simulink model "CompareBasisMRAC_knownDynamics_Obsolete"  (R2022b)
settings: Solver=ode4  StartTime=0.0  StopTime=30  FixedStep=1e-3  RelTol=1e-5  AbsTol=1e-7
values from neighbouring files (symbols this model uses):
  A = -1    [UniCenterMRAC.m]    (also in createPoints.m = []; greedySet2.m = []; runCompareBasisMRAC.m; runNewtonMRAC.m = -4)
  alpha0 = 0    [Run_Both_Model.m]    (also in Run_Deadzone.m; Run_ScalarModel.m; Slicing.m; UniCenterMRAC.m)
  Ar = -1    [UniCenterMRAC.m]    (also in runCompareBasisMRAC.m; runNewtonMRAC.m = -5; runTriggerTest.m = -10000; runVanDerPolTrigger.m = A)
  B = 1    [UniCenterMRAC.m]    (also in cholNP.m = A(kk:n,kk:n); cholwPiv.m = A(kk:n,kk:n); pivchol.m = A(kk:n,kk:n); runCompareBasisMRAC.m)
  beta0 = 0    [Run_Both_Model.m]    (also in Run_Deadzone.m; Run_ScalarModel.m; Slicing.m; UniCenterMRAC.m)
  Br = 1    [UniCenterMRAC.m]    (also in runCompareBasisMRAC.m; runNewtonMRAC.m; runTriggerTest.m; runVanDerPolTrigger.m = B)
  centers = linspace(-OmegaLim-ext,OmegaLim+ext,N)'    [UniCenterMRAC.m]    (also in getOfflineError.m = linspace(-OmegaLim-ext,OmegaLim+ext,Ns(nn))'; getOfflineErrorNewt.m = linspace(-OmegaLim-ext,OmegaLim+ext,Ns(nn))'; getOfflineErrorNewt2.m = linspace(-OmegaLim-ext,OmegaLim+ext,Ns(nn))'; getVDP_HNorm.m = omegaCover2(Ri,Ro,h(hh)))
  Dim = 1    [UniCenterMRAC.m]    (also in runCompareBasisMRAC.m; runNewtonMRAC.m; runTriggerTest.m; runWendlandMRAC.m)
  epsilon = powBound(nn)*norm_fs+delta    [UniCenterMRAC.m]    (also in runCompareBasisMRAC.m; runNewtonMRAC.m; runTriggerTest.m = PowerBound+delta; runVanDerPolTrigger.m = PowerBound*R+delta)
  fMag = 1    [UniCenterMRAC.m]    (also in runCompareBasisMRAC.m = 2; runNewtonMRAC.m; runTriggerTest.m = 2; runWendlandMRAC.m)
  ga = 10    [Run_Both_Model.m]    (also in Run_Deadzone.m; Run_ScalarModel.m; Slicing.m; UniCenterMRAC.m = 0)
  gb = 10    [Run_Both_Model.m]    (also in Run_Deadzone.m; Run_ScalarModel.m; Slicing.m; UniCenterMRAC.m = 0)
  gf = 10    [Run_Both_Model.m]    (also in Run_Deadzone.m; Run_ScalarModel.m; Slicing.m; UniCenterMRAC.m = 1)
  interps = linspace(-OmegaLim,OmegaLim,Ip)'    [UniCenterMRAC.m]    (also in runCompareBasisMRAC.m; runNewtonMRAC.m; runTriggerTest.m; runWendlandMRAC.m)
  K = kermat(centers,centers,type,par,scale)    [UniCenterMRAC.m]    (also in runCompareBasisMRAC.m; runNewtonMRAC.m; runTriggerTest.m; runVanDerPolTrigger.m = real(kermat(centers,centers,type,par,scale)))
  par = 1    [UniCenterMRAC.m]    (also in frbf.m = par-2; runCompareBasisMRAC.m; runNewtonMRAC.m; runTriggerTest.m)
  scale = 0.2    [UniCenterMRAC.m]    (also in runCompareBasisMRAC.m = 0.1; runNewtonMRAC.m = 0.5; runTriggerTest.m = 0.1; runVanDerPolTrigger.m = 0.3)
  sigma = 0.1    [Run_Both_Model.m]    (also in Run_Deadzone.m; Run_Project1i_haoran9.m; Run_ScalarModel.m; Slicing.m)
  SNU = 10    [UniCenterMRAC.m]    (also in runCompareBasisMRAC.m = 2; runNewtonMRAC.m; runTriggerTest.m = 2; runWendlandMRAC.m)
  StartMeasureTime = runTimes(tt)-1    [UniCenterMRAC.m]    (also in runCompareBasisMRAC.m = runTimes(tt)-10; runNewtonMRAC.m = runTimes(tt)-10; runTriggerTest.m = 0; runVanDerPolTrigger.m = 1990)
  targetCoefs = intmat\ySamps    [UniCenterMRAC.m]    (also in runCompareBasisMRAC.m; runNewtonMRAC.m; runTriggerTest.m; runWendlandMRAC.m)
  targetNu = 1/2*(sTarget+Dim/2)    (= 1.75)    [UniCenterMRAC.m]    (also in runCompareBasisMRAC.m; runNewtonMRAC.m; runTriggerTest.m; runWendlandMRAC.m)
  targetScale = 0.2    [UniCenterMRAC.m]    (also in runCompareBasisMRAC.m; runNewtonMRAC.m; runTriggerTest.m; runWendlandMRAC.m)
  V = zeros(fineN,fineN)    [UniCenterMRAC.m]    (also in getOfflineErrorNewt2.m = zeros(N,N); greedyCenters.m = ur(1:nn,index)'; greedySet.m = ur(1:nn,index)'; greedySet2.m = real(ur(1:nn,index)'))
  x0 = 0    [Run_Both_Model.m]    (also in Run_Deadzone.m; Run_Project1i_haoran9.m = 1; Run_ScalarModel.m; Slicing.m = 5)
  xr0 = 0    [Run_Both_Model.m]    (also in Run_Deadzone.m; Run_Project1i_haoran9.m; Run_ScalarModel.m; Slicing.m)
libraries: simulink x5
settings Model: Creator=owned  LastModifiedBy=Nathan
settings SolverCC: AlgebraicLoopSolver=TrustRegion
settings DebuggingCC: UnconnectedInputMsg=warning  UnconnectedOutputMsg=warning  UnconnectedLineMsg=warning  SFMachineParentedDataDiag=warning
settings ModelReferenceCC: EnableRefExpFcnMdlSchedulingChecks=on
settings RTWCC: DLArmComputeVersion=19.05

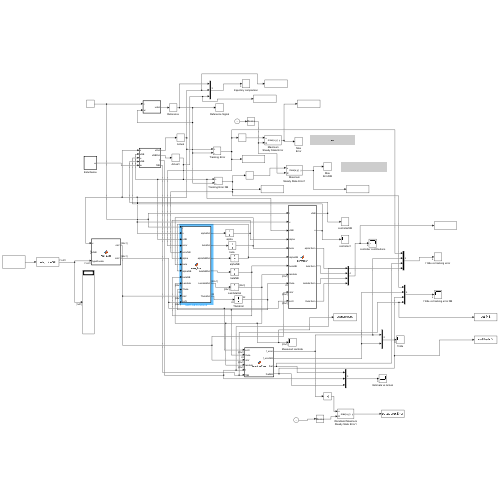
[thumbnail: Simulink's stored preview of the top-level diagram]
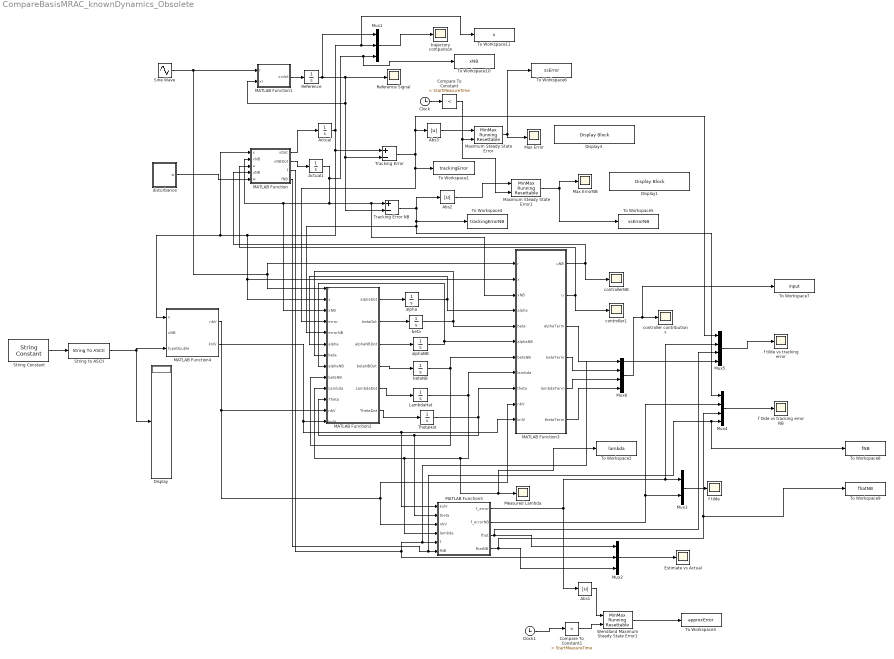
== system CompareBasisMRAC_knownDynamics_Obsolete ==
  " Maximum Steady State Error" : simulink/Math Operations/MinMax Running Resettable  Function=max  vinit=0.0
  " Maximum Steady State Error1" : simulink/Math Operations/MinMax Running Resettable  Function=max  vinit=0.0
  " Tracking Error" : Sum  Inputs=+-
  Abs1 : Abs  SaturateOnIntegerOverflow=off
  Abs2 : Abs  SaturateOnIntegerOverflow=off
  Abs3 : Abs  SaturateOnIntegerOverflow=off
  Actual : Integrator  InitialCondition=x0
  Actual1 : Integrator  InitialCondition=x0
  Clock : Clock
  Clock1 : Clock
  Compare To Constant : simulink/Logic and Bit Operations/Compare To Constant  relop=<  const=StartMeasureTime  OutDataTypeStr=boolean
  Compare To Constant1 : simulink/Logic and Bit Operations/Compare To Constant  relop=<  const=StartMeasureTime  OutDataTypeStr=boolean
  Display : Display
  Display1 : DisplayBlock  LabelPosition=Hide  Transparency=1
  Display3 : DisplayBlock  LabelPosition=Hide  Transparency=1
  Estimate vs Actual : Scope
  LambdaHat : Integrator
  MATLAB Function : MATLAB Function  TreatAsAtomicUnit=on
  MATLAB Function1 : MATLAB Function  TreatAsAtomicUnit=on
  MATLAB Function2 : MATLAB Function  TreatAsAtomicUnit=on
  MATLAB Function3 : MATLAB Function  TreatAsAtomicUnit=on
  MATLAB Function4 : MATLAB Function  TreatAsAtomicUnit=on
  MATLAB Function5 : MATLAB Function  TreatAsAtomicUnit=on
  Max Error : Scope
  Max ErrorNB : Scope
  Measured Lambda : Scope
  Mux1 : Mux  Inputs=3
  Mux2 : Mux  Inputs=3
  Mux3 : Mux  Inputs=2
  Mux4 : Mux
  Mux5 : Mux
  Mux6 : Mux
  Reference : Integrator  InitialCondition=xr0
  Reference Signal : Scope
  Sine Wave : Sin  Amplitude=SNU  Frequency=2*pi*0.1  SampleTime=0
  String Constant : StringConstant  String=type
  String to ASCII : StringToASCII
  ThetaHat : Integrator
  To Workspace1 : ToWorkspace  VariableName=trackingError  SaveFormat=Timeseries  SampleTime=-1
  To Workspace10 : ToWorkspace  VariableName=xNB  SaveFormat=Timeseries  SampleTime=-1
  To Workspace11 : ToWorkspace  VariableName=x  SaveFormat=Timeseries  SampleTime=-1
  To Workspace2 : ToWorkspace  VariableName=lambda  SaveFormat=Timeseries  SampleTime=-1
  To Workspace3 : ToWorkspace  VariableName=approxError  SaveFormat=Timeseries  SampleTime=-1
  To Workspace4 : ToWorkspace  VariableName=trackingErrorNB  SaveFormat=Timeseries  SampleTime=-1
  To Workspace5 : ToWorkspace  VariableName=ssErrorNB  SaveFormat=Timeseries  SampleTime=-1
  To Workspace6 : ToWorkspace  VariableName=ssError  SaveFormat=Timeseries  SampleTime=-1
  To Workspace7 : ToWorkspace  VariableName=input  SaveFormat=Timeseries  SampleTime=-1
  To Workspace8 : ToWorkspace  VariableName=fNB  SaveFormat=Timeseries  SampleTime=-1
  To Workspace9 : ToWorkspace  VariableName=fhatNB  SaveFormat=Timeseries  SampleTime=-1
  Tracking Error NB : Sum  Inputs=+-
  Wendland Maximum Steady State Error1 : simulink/Math Operations/MinMax Running Resettable  Function=max  vinit=0.0
  alpha : Integrator  InitialCondition=alpha0
  alphaNB : Integrator  InitialCondition=alpha0
  beta : Integrator  InitialCondition=beta0
  betaNB : Integrator  InitialCondition=beta0
  controller contributions : Scope
  controller1 : Scope
  controllerNB : Scope
  disturbance : MATLAB Function  TreatAsAtomicUnit=on
  f tilde : Scope
  f tilde vs tracking error : Scope
  f tilde vs tracking error NB : Scope
  trajectory comparison : Scope
  wires:
  Sine Wave/1 -> MATLAB Function1/1(r), MATLAB Function2/1(r), MATLAB Function3/1(r)
  MATLAB Function1/1(xrdot) -> Reference/1
  Reference/1 -> Tracking Error NB/2, " Tracking Error"/2, MATLAB Function1/2(xr), Reference Signal/1, Mux1/1
  MATLAB Function/1(xDot) -> Actual/1
  Actual/1 -> MATLAB Function/1(x), MATLAB Function4/1(x), MATLAB Function2/2(x), MATLAB Function3/2(x), " Tracking Error"/1, To Workspace11/1, Mux1/2
  " Tracking Error"/1 -> Mux5/1, Abs3/1, MATLAB Function2/4(error), To Workspace1/1
  MATLAB Function2/1(alphaDot) -> alpha/1
  MATLAB Function2/2(betaDot) -> beta/1
  MATLAB Function4/1(nbV) -> MATLAB Function5/3(nbV), MATLAB Function3/10(nbV), MATLAB Function2/12(nbV)
  alpha/1 -> MATLAB Function2/6(alpha), MATLAB Function3/4(alpha)
  beta/1 -> MATLAB Function2/7(beta), MATLAB Function3/5(beta)
  LambdaHat/1 -> MATLAB Function3/8(lambda), MATLAB Function5/4(lambda), MATLAB Function2/10(Lambda), To Workspace2/1, Measured Lambda/1
  MATLAB Function3/1(uNB) -> controllerNB/1, MATLAB Function/4(uNB)
  Clock/1 -> Compare To Constant/1
  Compare To Constant/1 -> " Maximum Steady State Error1"/2, " Maximum Steady State Error"/2
  " Maximum Steady State Error"/1 -> To Workspace6/1, Max Error/1
  Abs3/1 -> " Maximum Steady State Error"/1
  Mux1/1 -> trajectory comparison/1
  String Constant/1 -> String to ASCII/1
  String to ASCII/1 -> Display/1, MATLAB Function4/3(typeDouble)
  MATLAB Function5/1(f_error) -> Abs1/1, Mux5/2, Mux3/1
  Mux2/1 -> Estimate vs Actual/1
  MATLAB Function5/3(fhat) -> Mux5/3, Mux2/1
  Clock1/1 -> Compare To Constant1/1
  Abs1/1 -> Wendland Maximum Steady State Error1/1
  Compare To Constant1/1 -> Wendland Maximum Steady State Error1/2
  Wendland Maximum Steady State Error1/1 -> To Workspace3/1
  disturbance/1(w) -> MATLAB Function/5(w)
  MATLAB Function4/2(knlV) -> MATLAB Function5/1(knlV), MATLAB Function3/11(knlV), MATLAB Function2/13(knlV)
  MATLAB Function2/5(LambdaDot) -> LambdaHat/1
  MATLAB Function2/6(ThetaDot) -> ThetaHat/1
  ThetaHat/1 -> MATLAB Function3/9(theta), MATLAB Function5/2(theta), MATLAB Function2/11(Theta)
  MATLAB Function3/2(u) -> MATLAB Function/3(u), controller1/1
  MATLAB Function/2(xNBDot) -> Actual1/1
  Actual1/1 -> To Workspace10/1, Mux1/3, MATLAB Function3/3(xNB), Tracking Error NB/1, MATLAB Function2/3(xNB), MATLAB Function/2(xNB)
  MATLAB Function2/4(betaNBDot) -> betaNB/1
  betaNB/1 -> MATLAB Function2/9(betaNB), MATLAB Function3/7(betaNB)
  MATLAB Function2/3(alphaNBDot) -> alphaNB/1
  alphaNB/1 -> MATLAB Function2/8(alphaNB), MATLAB Function3/6(alphaNB)
  Tracking Error NB/1 -> To Workspace4/1, Mux4/1, MATLAB Function2/5(errorNB), Abs2/1
  Abs2/1 -> " Maximum Steady State Error1"/1
  " Maximum Steady State Error1"/1 -> To Workspace5/1, Max ErrorNB/1
  MATLAB Function5/4(fhatNB) -> To Workspace9/1, Mux4/3, Mux2/3
  MATLAB Function5/2(f_errorNB) -> Mux4/2, Mux3/2
  MATLAB Function/3(f) -> Mux2/2, Mux5/4, MATLAB Function5/5(f)
  MATLAB Function/4(fNB) -> To Workspace8/1, Mux4/4, MATLAB Function5/6(fNB)
  Mux3/1 -> f tilde/1
  Mux4/1 -> f tilde vs tracking error NB/1
  Mux5/1 -> f tilde vs tracking error/1
  MATLAB Function3/3(alphaTerm) -> Mux6/1
  MATLAB Function3/4(betaTerm) -> Mux6/2
  MATLAB Function3/5(lambdaTerm) -> Mux6/3
  MATLAB Function3/6(thetaTerm) -> Mux6/4
  Mux6/1 -> To Workspace7/1, controller contributions/1

== matlab function CompareBasisMRAC_knownDynamics_Obsolete/MATLAB Function3 ==
  data: r input; x input; xNB input; alpha input; beta input; alphaNB input; betaNB input; lambda input size=[N 1]; theta input size=[N 1]; nbV input; knlV input; uNB output size=1; epsilon parameter; B parameter; u output; alphaTerm output; betaTerm output; lambdaTerm output; thetaTerm output
function [uNB,u,alphaTerm,betaTerm,lambdaTerm,thetaTerm] = controller(r, x,xNB, alpha,beta,alphaNB,betaNB, lambda,theta, nbV,knlV,epsilon,B)
% P= 1;
% if B*P*x >= 0
%     vN = epsilon;
% else
%     vN = -epsilon;
% end
% u = alpha*x+beta*r+theta'*knlV;
% uNB = alphaNB*xNB+betaNB*r+lambda'*nbV;


u = r + theta'*knlV;
uNB = r + lambda'*nbV;

alphaTerm = alphaNB*xNB;
betaTerm = betaNB*r;
lambdaTerm = lambda'*nbV;
thetaTerm = theta'*knlV;
end

== matlab function CompareBasisMRAC_knownDynamics_Obsolete/MATLAB Function4 ==
  data: x input; xNB input; centers parameter; typeDouble input; nbV output; scale parameter; par parameter; knlV output; K parameter; V parameter
function [nbV,knlV]  = Knl_Eval(x,xNB,centers,typeDouble, scale, par,K,V)
    type = char(typeDouble(typeDouble~=0));
    knlV = real(kermat(centers,x,type,par,scale));
    knlVNB = real(kermat(centers,xNB,type,par,scale));
    N = length(centers);
    z = diag(K);
    v_x = zeros(N,1);
    P = sqrt(K(1,1));

    v_x(1) = knlVNB(1)/P;
%     
%     V = zeros(N,N);
%     if N > 1
%         V(:,1) = K(:,1)/P;
%         w = V(:,1).^2;
%         NN = V(2,:)*v_x;
%         P = sqrt(z(2)-w(2));
%         
%         for jj = 1:N-1
%             e = zeros(N,1);
%             e(jj+1) = 1;
%             Vm = V(:,1:jj);
%             u = K*e-Vm*Vm'*e;
%             u_x = knlV(jj+1) - NN;
%             v_x(jj+1) = u_x/P; % Newton Basis evaluated at x
%             V(:,jj+1) = u/P; % Newton Basis evaluated at the centers
%             w = V(:,jj+1).^2 + w; % Updating sum of Newton basis squared at the centers
%             if jj ~=N-1
%                 NN = V(jj+2,:)*v_x;
%                 P = sqrt(z(jj+2)-w(jj+2));
%             end
%         end
%     end
%     nbV = v_x;

    
    if N > 1
        w = V(1:N,1).^2;
        NN = V(2,1:N)*v_x;
        P = sqrt(z(2)-w(2));
        
        for jj = 1:N-1
            u_x = knlVNB(jj+1) - NN;
            v_x(jj+1) = u_x/P; % Newton Basis evaluated at x
            w = V(1:N,jj+1).^2 + w; % Updating sum of Newton basis squared at the centers
            if jj ~=N-1
                NN = V(jj+2,1:N)*v_x;
                P = sqrt(z(jj+2)-w(jj+2));
            end
        end
    end
    nbV = v_x;


end

== matlab function CompareBasisMRAC_knownDynamics_Obsolete/MATLAB Function5 ==
  data: knlV input; theta input; nbV input; f_error output size=1; f_errorNB output; lambda input; f input; fhat output; fhatNB output; fNB input
function [f_error,f_errorNB,fhat,fhatNB]  = functionError(knlV,theta,nbV,lambda, f,fNB)
fhatNB = lambda'*nbV;
f_errorNB = fNB-fhatNB;

fhat = theta'*knlV;
f_error = f-fhat;

== matlab function CompareBasisMRAC_knownDynamics_Obsolete/disturbance ==
  data: w output; delta parameter
function w   = plant(delta)
% 
w = 0.5*rand;

== matlab function CompareBasisMRAC_knownDynamics_Obsolete/MATLAB Function1 ==
  data: r input; xr input; xrdot output; Ar parameter; Br parameter
function xrdot = reference(r,xr,Ar, Br)

xrdot = Ar*xr+Br*r;

== matlab function CompareBasisMRAC_knownDynamics_Obsolete/MATLAB Function ==
  data: x input; xNB input; u input; uNB input; A parameter; B parameter; w input; interps parameter; targetCoefs parameter; xDot output; xNBDot output; targetScale parameter; targetNu parameter; Dim parameter; f output; fNB output; fMag parameter
function [xDot,xNBDot,f,fNB]  = plant(x,xNB,u,uNB,A, B,w,interps, targetCoefs,targetScale,targetNu, Dim,fMag)
% 
% targetKnlV = real(kermat(interps,x,'ms',targetNu-Dim/2,targetScale));
% f = targetCoefs'*targetKnlV;

f = fMag*tanh(0.1*x);

% targetKnlV_NB = real(kermat(interps,xNB,'ms',targetNu-Dim/2,targetScale));
% fNB = targetCoefs'*targetKnlV_NB;

fNB = fMag*tanh(0.1*xNB);


xDot = A*x+B*(u+f+w);
xNBDot = A*xNB+B*(uNB+fNB+w);

== matlab function CompareBasisMRAC_knownDynamics_Obsolete/MATLAB Function2 ==
  data: ga parameter; gb parameter; gf parameter; sigma parameter; alphaDot output size=1; betaDot output size=1; alphaNBDot output; betaNBDot output; LambdaDot output; ThetaDot output size=N; r input; x input; xNB input; error input; errorNB input; alpha input; beta input; alphaNB input; betaNB input; Lambda input; Theta input; nbV input size=[N,1]; knlV input size=[N 1]; epsilon parameter; K parameter
function [alphaDot, betaDot,alphaNBDot, betaNBDot, LambdaDot, ThetaDot] = evo_law(ga, gb, gf, sigma, r, x, xNB, error,errorNB, alpha, beta,alphaNB, betaNB, Lambda, Theta, nbV,knlV,epsilon, K)


%% Standard RKHS Sigma Mod
% alphaDot=-ga*x*error-sigma*alpha;
% betaDot=-gb*r*error-sigma*beta;
% ThetaDot=gf*invK*knlV*error-sigma*Theta;

%% Standard RKHS Deadzone
if abs(error) > epsilon
    alphaDot=-ga*x*error;
    betaDot=-gb*r*error;
    ThetaDot=-gf*K\knlV*error;
else
    alphaDot=0;
    betaDot=0;
    ThetaDot=zeros(size(nbV));
end

if abs(errorNB) > epsilon
    alphaNBDot=-ga*xNB*errorNB;
    betaNBDot=-gb*r*errorNB;
    LambdaDot=-1/gf*nbV*errorNB;
else
    alphaNBDot=0;
    betaNBDot=0;
    LambdaDot=zeros(size(nbV));
end




%% Standard RKHS Deadzone
% if abs(error)>epsilon
%     alphaDot=-ga*x*error;
%     betaDot=-gb*r*error;
%     ThetaDot=gf*K\knlV*error;
% else
%     alphaDot=0;
%     betaDot=0;
%     ThetaDot=zeros(size(knlV));
% end
